simulink model "FLC_sim_pulse"  (R2023a)
settings: Solver=VariableStepAuto  StartTime=0.0  StopTime=16.0  RelTol=1e-3
libraries: fuzblock x1, SignalEditorBlockLib x1
settings Model: Creator=dimal  LastModifiedBy=dimal

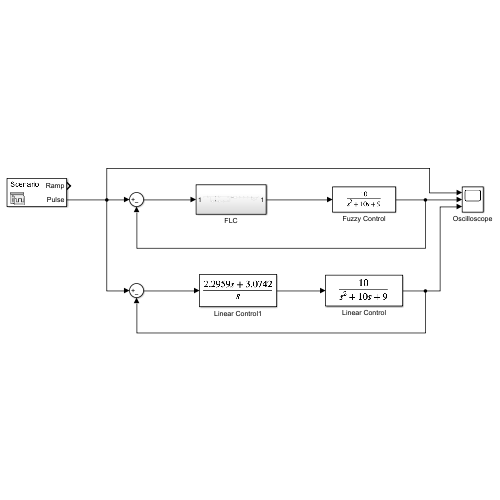
[thumbnail: Simulink's stored preview of the top-level diagram]
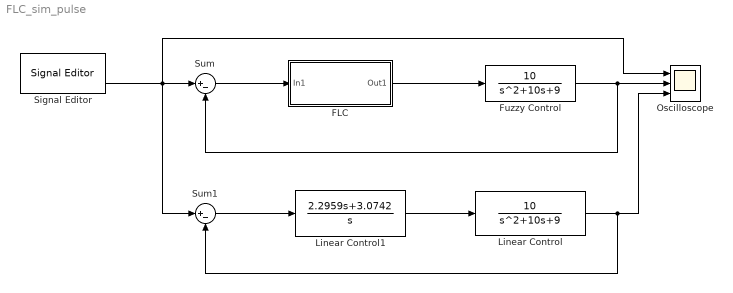
== system FLC_sim_pulse ==
  FLC : Subsystem
  Fuzzy Control : TransferFcn  Numerator=[10]  Denominator=[1 10 9]
  Linear Control : TransferFcn  Numerator=[10]  Denominator=[1 10 9]
  Linear Control1 : TransferFcn  Numerator=[2.2959 3.0742]  Denominator=[1 0]
  Oscilloscope : Scope  NumInputPorts=3
  Signal Editor : SignalEditorBlockLib/Signal Editor  FileName=singal.mat  ActiveScenario=Scenario  ActiveSignal=Pulse  IsBus=off  OutputBusObjectStr=Bus: BusObject  SampleTime=0.01  OutputAfterFinalValue=Setting to zero  Unit=inherit  PreserveSignalName=on  ApplySigPropsToAllScenarios=on
  Sum : Sum  Inputs=|+-
  Sum1 : Sum  Inputs=|+-
  wires:
  FLC/1(Out1) -> Fuzzy Control/1
  Sum/1 -> FLC/1(In1)
  Signal Editor/2 -> Sum1/1, Oscilloscope/1, Sum/1
  Fuzzy Control/1 -> Sum/2, Oscilloscope/2
  Sum1/1 -> Linear Control1/1
  Linear Control1/1 -> Linear Control/1
  Linear Control/1 -> Oscilloscope/3, Sum1/2

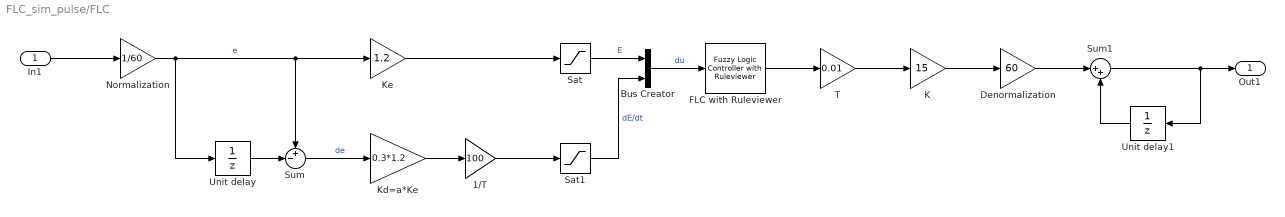
== system FLC_sim_pulse/FLC ==
  In1 : Inport
  1/T : Gain  Gain=100
  Bus Creator : BusCreator  Inputs=2
  Denormalization : Gain  Gain=60
  FLC with Ruleviewer : fuzblock/Fuzzy Logic  Controller  with Ruleviewer  fismatrix=FLC  Ts=2
  K : Gain  Gain=15
  Kd=a*Ke : Gain  Gain=0.3*1.2
  Ke : Gain  Gain=1.2
  Normalization : Gain  Gain=1/60
  Sat : Saturate
  Sat1 : Saturate
  Sum : Sum  Inputs=+-|
  Sum1 : Sum  Inputs=|++
  T : Gain  Gain=0.01
  Unit delay : UnitDelay  SampleTime=-1  HasFrameUpgradeWarning=on
  Unit delay1 : UnitDelay  SampleTime=-1  HasFrameUpgradeWarning=on
  Out1 : Outport
  wires:
  Normalization/1 -> Unit delay/1, Sum/1, Ke/1  "e"
  Ke/1 -> Sat/1
  Sum/1 -> Kd=a*Ke/1  "de"
  Kd=a*Ke/1 -> 1/T/1
  1/T/1 -> Sat1/1
  Sat/1 -> Bus Creator/1  "E"
  Sat1/1 -> Bus Creator/2  "dE/dt"
  FLC with Ruleviewer/1 -> T/1
  T/1 -> K/1
  K/1 -> Denormalization/1
  Denormalization/1 -> Sum1/1
  Unit delay/1 -> Sum/2
  Sum1/1 -> Out1/1, Unit delay1/1
  Unit delay1/1 -> Sum1/2
  In1/1 -> Normalization/1
  Bus Creator/1 -> FLC with Ruleviewer/1  "du"
